simulink model "testdone"  (R2024b)
settings: Solver=VariableStepAuto  StartTime=0.0  StopTime=1.0  RelTol=1e-3
libraries: spsSeriesRLCBranchLib x4, spsVoltageMeasurementLib x4, spsUniversalBridgeLib x2, spsDCMachineLib x1, spsDCVoltageSourceLib x1, spsThreePhaseSourceLib x1, sps_lib x1

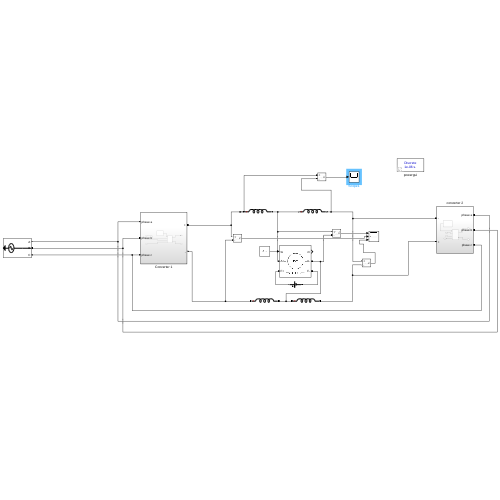
[thumbnail: Simulink's stored preview of the top-level diagram]
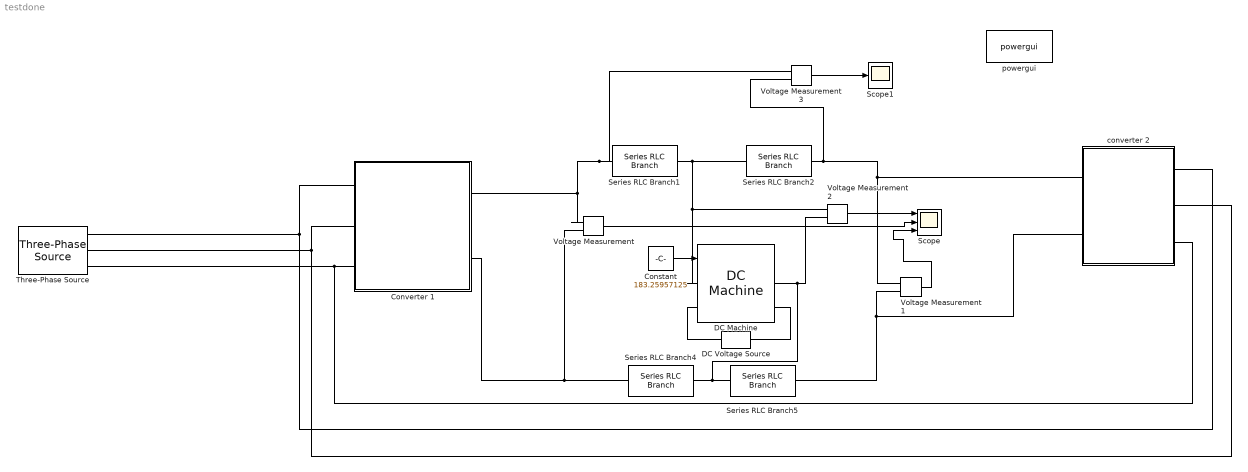
== system testdone ==
  Constant : Constant  Value=183.25957125
  Converter 1 : Subsystem
  DC Machine : spsDCMachineLib/DC Machine  PresetModel=01: 5HP 240V 1750RPM Field:300V  MechanicalLoad=Speed w  FieldType=Wound  ShowDetailedParameters=on  MeasurementBus=off  RLa=[2.581 0.028]  RLf=[281.2 156]  Laf=0.9483  MachineConstant=Torque constant (N.m/A)  Ke=1.8  Kt=1.8  J=0.02215  Bm=0.002953  Tf=0.5161  w0=1  Ifinit=1.06685633001422  TsPowergui=0  TsBlock=-1
  DC Voltage Source : spsDCVoltageSourceLib/DC Voltage Source  Amplitude=300  Measurements=None
  Scope : Scope  NumInputPorts=3
  Scope1 : Scope
  Series RLC Branch{1..2,4..5} (4 alike) : spsSeriesRLCBranchLib/Series RLC Branch  LConnTagsString=__new0  RConnTagsString=__new0  BranchType=L  Resistance=100  Inductance=0.083  SetiL0=off  InitialCurrent=0  Capacitance=1e-6  Setx0=off  InitialVoltage=0  Measurements=None
  Three-Phase Source : spsThreePhaseSourceLib/Three-Phase Source  InternalConnection=Yg  VoltagePhases=off  Voltage=230*sqrt(3)  PhaseAngle=0  Voltage_phases=[25e3 25e3 25e3]/sqrt(3)  PhaseAngles_phases=[0 -120 +120]  Frequency=50  NonIdealSource=off  SpecifyImpedance=off  Resistance=0.8929  Inductance=16.58e-3  ShortCircuitLevel=100e6  BaseVoltage=25e3  XRratio=7  BusType=swing  Pref=10e3  Qref=0  Prefabc=[10e3, 10e3, 10e3]  Qrefabc=[0, 0, 0]  Qmin=-inf  Qmax=inf
  Voltage Measurement{,1..3} (4 alike) : spsVoltageMeasurementLib/Voltage Measurement  PhasorSimulation=off  OutputType=Complex  PSBequivalent=0
  converter 2 : Subsystem
  powergui : sps_lib/powergui  Priority=1  SimulationMode=Discrete  SampleTime=1e-6  frequency=60  Iterations=50  frequencyindice=0  Pbase=100e6  ErrMax=1e-4  UnitsV=kV  UnitsW=MW  buscounter=0  FunctionMessages=off  echomessages=off  EnableUseOfTLC=off  CurrentSourceSwitches=off  DisableSnubberDevices=off  DisableRonSwitches=off  DisableVfSwitches=off  DisplayEquations=off  AutomaticDiscreteSolvers=off  SolverType=Tustin/Backward Euler (TBE)  Interpol=off  ExternalGateDelay=off  methode=off  Ts=100  x0status=blocks  SPID=on  SwTol=0  HookPort=off  NonlinearTolerance=1e-4  nMaxIteration=100  ContinueOnMaxIteration=off  RestoreLinks=warning  ResistiveCurrentMeasurement=off  Frange=[0:2:500]  Ylog=off  Xlog=on  ShowGrid=off  save=off  variable=ZData  structure=0  ZoomFFT=off  StartTime=0.0  cycles=1  DisplayStyle=1  fundamental=60  FreqAxis=off  MaxFrequency=1000  frequencyindicesteady=1  RmsSteady=1  display=off
  wires:
  Voltage Measurement1/1 -> Scope/3
  Voltage Measurement2/1 -> Scope/1
  Voltage Measurement3/1 -> Scope1/1
  Constant/1 -> DC Machine/1
  Voltage Measurement/1 -> Scope/2
  connections:
  Voltage Measurement/LConn1 -- Series RLC Branch1/LConn1 -- Voltage Measurement3/LConn1 -- Converter 1/RConn1
  Series RLC Branch4/RConn1 -- Series RLC Branch5/LConn1 -- Voltage Measurement2/LConn2 -- DC Machine/RConn1
  converter 2/LConn2 -- Converter 1/LConn2 -- Three-Phase Source/RConn2
  Converter 1/RConn2 -- Voltage Measurement/LConn2 -- Series RLC Branch4/LConn1
  Three-Phase Source/RConn3 -- Converter 1/LConn3 -- converter 2/LConn3
  Series RLC Branch1/RConn1 -- Series RLC Branch2/LConn1 -- Voltage Measurement2/LConn1 -- DC Machine/LConn1
  converter 2/RConn2 -- Voltage Measurement1/LConn2 -- Series RLC Branch5/RConn1
  converter 2/LConn1 -- Converter 1/LConn1 -- Three-Phase Source/RConn1
  Series RLC Branch2/RConn1 -- Voltage Measurement3/LConn2 -- Voltage Measurement1/LConn1 -- converter 2/RConn1
  DC Voltage Source/RConn1 -- DC Machine/LConn2
  DC Voltage Source/LConn1 -- DC Machine/RConn2

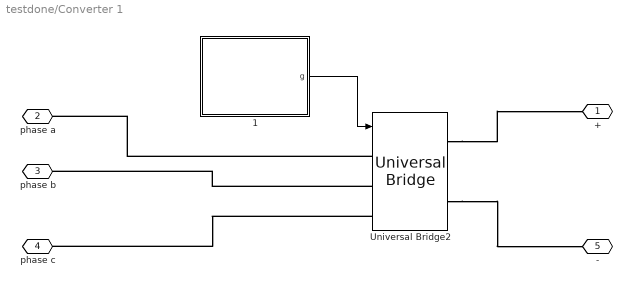
== system testdone/Converter 1 ==
  1 : Subsystem
  Universal Bridge2 : spsUniversalBridgeLib/Universal Bridge  Arms=3  SnubberResistance=1e5  SnubberCapacitance=inf  Device=Thyristors  Ron=1e-5  Lon=0  ForwardVoltages="[  0  0  ]"  ForwardVoltage=0  GTOparameters=[ 10e-6 , 20e-6 ]  IGBTparameters=[ 1e-6 , 2e-6 ]  Measurements=None  Measurements_2=None  converterType=Rectifier
  + : PMIOPort  Side=Right
  phase a : PMIOPort  Port=2  Side=Left
  phase b : PMIOPort  Port=3  Side=Left
  phase c : PMIOPort  Port=4  Side=Left
  - : PMIOPort  Port=5  Side=Right
  wires:
  1/1(g) -> Universal Bridge2/1
  connections:
  Universal Bridge2/RConn2 -- -/RConn1
  Universal Bridge2/RConn1 -- +/RConn1
  Universal Bridge2/LConn1 -- phase a/RConn1
  Universal Bridge2/LConn3 -- phase c/RConn1
  Universal Bridge2/LConn2 -- phase b/RConn1

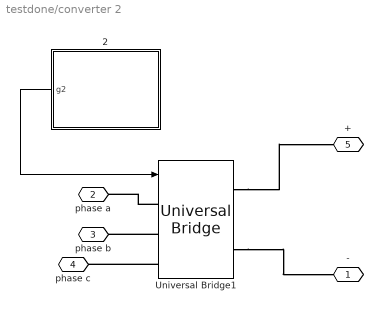
== system testdone/converter 2 ==
  2 : Subsystem
  Universal Bridge1 : spsUniversalBridgeLib/Universal Bridge  Arms=3  SnubberResistance=1e5  SnubberCapacitance=inf  Device=Thyristors  Ron=1e-5  Lon=0  ForwardVoltages="[  0  0  ]"  ForwardVoltage=0  GTOparameters=[ 10e-6 , 20e-6 ]  IGBTparameters=[ 1e-6 , 2e-6 ]  Measurements=None  Measurements_2=None  converterType=Rectifier
  - : PMIOPort  Side=Right
  phase a : PMIOPort  Port=2  Side=Left
  phase b : PMIOPort  Port=3  Side=Left
  phase c : PMIOPort  Port=4  Side=Left
  + : PMIOPort  Port=5  Side=Right
  wires:
  2/1(g2) -> Universal Bridge1/1
  connections:
  Universal Bridge1/LConn2 -- phase b/RConn1
  Universal Bridge1/LConn3 -- phase c/RConn1
  Universal Bridge1/LConn1 -- phase a/RConn1
  Universal Bridge1/RConn1 -- +/RConn1
  Universal Bridge1/RConn2 -- -/RConn1

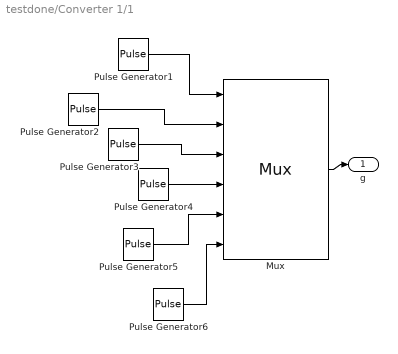
== system testdone/Converter 1/1 ==
  Mux : Mux  Inputs=6
  Pulse Generator1 : DiscretePulseGenerator  PulseType=Time based  Period=0.02  PulseWidth=14  PhaseDelay=(1/6)*(1/50)
  Pulse Generator2 : DiscretePulseGenerator  PulseType=Time based  Period=0.02  PulseWidth=14  PhaseDelay=(2/6)*(1/50)
  Pulse Generator3 : DiscretePulseGenerator  PulseType=Time based  Period=0.02  PulseWidth=14  PhaseDelay=(3/6)*(1/50)
  Pulse Generator4 : DiscretePulseGenerator  PulseType=Time based  Period=0.02  PulseWidth=14  PhaseDelay=(4/6)*(1/50)
  Pulse Generator5 : DiscretePulseGenerator  PulseType=Time based  Period=0.02  PulseWidth=14  PhaseDelay=(5/6)*(1/50)
  Pulse Generator6 : DiscretePulseGenerator  PulseType=Time based  Period=0.02  PulseWidth=14  PhaseDelay=1/50
  g : Outport  VectorParamsAs1DForOutWhenUnconnected=off
  wires:
  Pulse Generator1/1 -> Mux/1
  Pulse Generator5/1 -> Mux/5
  Pulse Generator6/1 -> Mux/6
  Pulse Generator3/1 -> Mux/3
  Mux/1 -> g/1
  Pulse Generator4/1 -> Mux/4
  Pulse Generator2/1 -> Mux/2

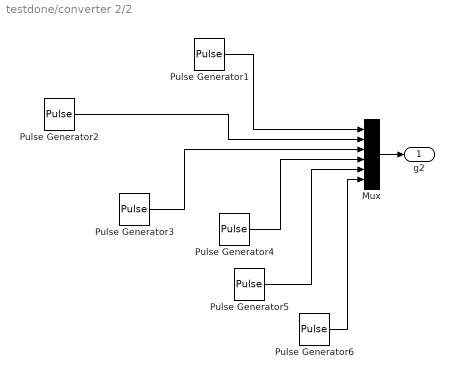
== system testdone/converter 2/2 ==
  Mux : Mux  Inputs=6
  Pulse Generator1 : DiscretePulseGenerator  PulseType=Time based  Period=0.02  PulseWidth=14  PhaseDelay=(3/6)*(1/50)
  Pulse Generator2 : DiscretePulseGenerator  PulseType=Time based  Period=0.02  PulseWidth=14  PhaseDelay=(4/6)*(1/50)
  Pulse Generator3 : DiscretePulseGenerator  PulseType=Time based  Period=0.02  PulseWidth=14  PhaseDelay=(5/6)*(1/50)
  Pulse Generator4 : DiscretePulseGenerator  PulseType=Time based  Period=0.02  PulseWidth=14  PhaseDelay=(1/50)
  Pulse Generator5 : DiscretePulseGenerator  PulseType=Time based  Period=0.02  PulseWidth=14  PhaseDelay=(1/50)*(7/6)
  Pulse Generator6 : DiscretePulseGenerator  PulseType=Time based  Period=0.02  PulseWidth=14  PhaseDelay=(1/50)*(8/6)
  g2 : Outport  VectorParamsAs1DForOutWhenUnconnected=off
  wires:
  Pulse Generator2/1 -> Mux/2
  Pulse Generator4/1 -> Mux/4
  Mux/1 -> g2/1
  Pulse Generator3/1 -> Mux/3
  Pulse Generator6/1 -> Mux/6
  Pulse Generator5/1 -> Mux/5
  Pulse Generator1/1 -> Mux/1
